simulink library "Servomotor_Lib"  (R2020a)
settings: Solver=VariableStepAuto  StartTime=0.0  StopTime=10.0  RelTol=1e-3
undefined symbols (not defined in the file): Servomotor, WT_Params, X, Y, Yaw_System_Lib, Z
libraries: fl_lib x51, nesl_utility x20, sdl_lib x20, ee_lib x8, sm_lib x4, Yaw_Actuation_Lib x1
(part 2 of 2)

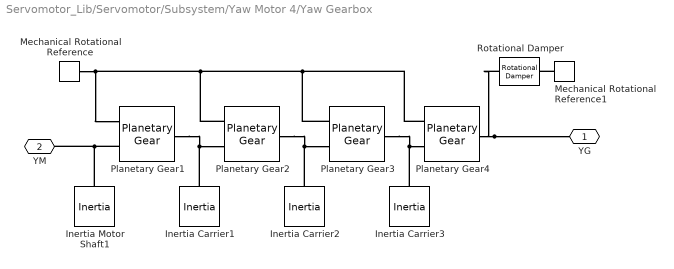
== system Servomotor_Lib/Servomotor/Subsystem/Yaw Motor 4/Yaw Gearbox ==
  Inertia Carrier1 : fl_lib/Mechanical/Rotational Elements/Inertia  inertia=WT_Params.Yaw_Actuator.inertia_carrier kg*m^2  w_specify=off  w_priority=High  w=0 rad/s  w_nominal_specify=off  w_nominal_unit=rad/s  w_nominal_value=1  t_specify=off  t_priority=None  t=0 N*m  t_nominal_specify=off  t_nominal_unit=N*m  t_nominal_value=1
  Inertia Carrier2 : fl_lib/Mechanical/Rotational Elements/Inertia  inertia=WT_Params.Yaw_Actuator.inertia_carrier kg*m^2  w_specify=off  w_priority=High  w=0 rad/s  w_nominal_specify=off  w_nominal_unit=rad/s  w_nominal_value=1  t_specify=off  t_priority=None  t=0 N*m  t_nominal_specify=off  t_nominal_unit=N*m  t_nominal_value=1
  Inertia Carrier3 : fl_lib/Mechanical/Rotational Elements/Inertia  inertia=WT_Params.Yaw_Actuator.inertia_carrier kg*m^2  w_specify=off  w_priority=High  w=0 rad/s  w_nominal_specify=off  w_nominal_unit=rad/s  w_nominal_value=1  t_specify=off  t_priority=None  t=0 N*m  t_nominal_specify=off  t_nominal_unit=N*m  t_nominal_value=1
  Inertia Motor Shaft1 : fl_lib/Mechanical/Rotational Elements/Inertia  inertia=WT_Params.Yaw_Actuator.inertia_motor_shaft kg*m^2  w_specify=off  w_priority=High  w=0 rad/s  w_nominal_specify=off  w_nominal_unit=rad/s  w_nominal_value=1  t_specify=off  t_priority=None  t=0 N*m  t_nominal_specify=off  t_nominal_unit=N*m  t_nominal_value=1
  Mechanical Rotational Reference : fl_lib/Mechanical/Rotational Elements/Mechanical Rotational Reference
  Mechanical Rotational Reference1 : fl_lib/Mechanical/Rotational Elements/Mechanical Rotational Reference
  Planetary Gear1 : sdl_lib/Gears/Planetary Gear  rs_ratio=WT_Params.Yaw_Actuator.p_gear_rato_step_1-1  friction_model=sdl.enum.gear_friction.none  mu_visc=[0, 0] N*m/(rad/s)  efficiency=[.96, .98]  temperature_TLU=[280, 300, 320] K  efficiency_sp_TLU=[.95, .9, .85]  efficiency_rp_TLU=[.95, .9, .85]  pwr_thr=[.001, .001] W  thermal_mass=50 J/K  T_init=300 K  model_inertia=simscape.enum.onoff.off  planet_inertia=0.001 kg*m^2
      settings: SourceProductBaseCode=LD
  Planetary Gear2 : sdl_lib/Gears/Planetary Gear  rs_ratio=WT_Params.Yaw_Actuator.p_gear_rato_step_2-1  friction_model=sdl.enum.gear_friction.none  mu_visc=[0, 0] N*m/(rad/s)  efficiency=[.96, .98]  temperature_TLU=[280, 300, 320] K  efficiency_sp_TLU=[.95, .9, .85]  efficiency_rp_TLU=[.95, .9, .85]  pwr_thr=[.001, .001] W  thermal_mass=50 J/K  T_init=300 K  model_inertia=simscape.enum.onoff.off  planet_inertia=0.001 kg*m^2
      settings: SourceProductBaseCode=LD
  Planetary Gear3 : sdl_lib/Gears/Planetary Gear  rs_ratio=WT_Params.Yaw_Actuator.p_gear_rato_step_3-1  friction_model=sdl.enum.gear_friction.none  mu_visc=[0, 0] N*m/(rad/s)  efficiency=[.96, .98]  temperature_TLU=[280, 300, 320] K  efficiency_sp_TLU=[.95, .9, .85]  efficiency_rp_TLU=[.95, .9, .85]  pwr_thr=[.001, .001] W  thermal_mass=50 J/K  T_init=300 K  model_inertia=simscape.enum.onoff.off  planet_inertia=0.001 kg*m^2
      settings: SourceProductBaseCode=LD
  Planetary Gear4 : sdl_lib/Gears/Planetary Gear  rs_ratio=WT_Params.Yaw_Actuator.p_gear_rato_step_4-1  friction_model=sdl.enum.gear_friction.none  mu_visc=[0, 0] N*m/(rad/s)  efficiency=[.96, .98]  temperature_TLU=[280, 300, 320] K  efficiency_sp_TLU=[.95, .9, .85]  efficiency_rp_TLU=[.95, .9, .85]  pwr_thr=[.001, .001] W  thermal_mass=50 J/K  T_init=300 K  model_inertia=simscape.enum.onoff.off  planet_inertia=0.001 kg*m^2
      settings: SourceProductBaseCode=LD
  Rotational Damper : fl_lib/Mechanical/Rotational Elements/Rotational Damper  D=WT_Params.Yaw_Actuator.damping N*m/(rad/s)  w_specify=off  w_priority=None  w=0 rad/s  w_nominal_specify=off  w_nominal_unit=rad/s  w_nominal_value=1  t_specify=off  t_priority=None  t=0 N*m  t_nominal_specify=off  t_nominal_unit=N*m  t_nominal_value=1
  YG : PMIOPort  Side=Right
  "YM " : PMIOPort  Port=2  Side=Left
  connections:
  Planetary Gear2/LConn1 -- Inertia Carrier2/LConn1 -- Planetary Gear3/RConn2
  Planetary Gear4/LConn1 -- Rotational Damper/LConn1 -- YG/RConn1
  Mechanical Rotational Reference1/LConn1 -- Rotational Damper/RConn1
  Planetary Gear4/RConn1 -- Planetary Gear3/RConn1 -- Mechanical Rotational Reference/LConn1 -- Planetary Gear1/RConn1 -- Planetary Gear2/RConn1
  Planetary Gear3/LConn1 -- Inertia Carrier3/LConn1 -- Planetary Gear4/RConn2
  Planetary Gear1/RConn2 -- "YM "/RConn1 -- Inertia Motor Shaft1/LConn1
  Planetary Gear1/LConn1 -- Inertia Carrier1/LConn1 -- Planetary Gear2/RConn2
